simulink model "NLMPC_Acado_Deploy_Speedgoat"  (R2021b)
settings: Solver=ode4  StartTime=0.0  StopTime=250  FixedStep=Ts  RelTol=1e-3  EnableMultiTasking=on
InitFcn:
  | ts = 0.001;
  | sin_base_freq = 1;
  | ampl = 6;
values from neighbouring files (symbols this model uses):
  Ad = sysd.A    [ACADO_NMPC_Main_File.m]
  Bd = sysd.B    [ACADO_NMPC_Main_File.m]
  eta = 0.94    [ACADO_NMPC_Main_File.m]
  Fext = [0 -1808.57139 -3027.52429 -3695.96924 -3861.91987 -3579.58608 -2906.76949 -1902.55612 -625.46835 867.809323 2523.07436 4288.62667 ... (9001 elements, 9001x1)]    [Fext.mat]
  Fk = 13893.63    [ACADO_NMPC_Main_File.m]
  Ts = 0.1    [ACADO_NMPC_Main_File.m]
  Wh1 = 2*[0         0      -c11/2   0 ... (first row only)    [ACADO_NMPC_Main_File.m]
  Wh2 = 2*[0         0       0       0 ... (first row only)    [ACADO_NMPC_Main_File.m]
  Wh3 = 2*[0         0       0       0 ... (first row only)    [ACADO_NMPC_Main_File.m]
  Wh4 = 2*[0         0      -c11/2   0 ... (first row only)    [ACADO_NMPC_Main_File.m]
  WNmat = WN    [ACADO_NMPC_Main_File.m]
  yref = [y(:);yN(:)]    [ACADO_NMPC_Main_File.m]
undefined symbols (not defined in the file or in its folder): C, IO, Mode
libraries: simulink x1, speedgoatlib_IO754 x1, dspstat3 x1
settings Model: sg_rtwmakecfg_data=_sglibc__sg_netxLib_  Creator=lab  LastModifiedBy=z4q9r
settings SolverCC: ConcurrentTasks=on  AlgebraicLoopSolver=TrustRegion  PositivePriorityOrder=on  AutoInsertRateTranBlk=on  InsertRTBMode=Never (minimum delay)
settings DataIOCC: LimitDataPoints=on  SaveFormat=StructureWithTime  ReturnWorkspaceOutputs=off
settings OptimizationCC: BlockReduction=off  DefaultParameterBehavior=Inlined  OptimizeBlockIOStorage=off  BufferReuse=off  GlobalBufferReuse=off  ExpressionFolding=off  LocalBlockOutputs=off  OptimizeDataStoreBuffers=off  BusAssignmentInplaceUpdate=off
settings DebuggingCC: TasksWithSamePriorityMsg=none  UnconnectedInputMsg=none  UnconnectedOutputMsg=none  UnconnectedLineMsg=none  SFMachineParentedDataDiag=warning  ArithmeticOperatorsInVariantConditions=warning
settings HardwareCC: ProdBitPerLong=64  ProdLongLongMode=on  ProdHWDeviceType=Intel->x86-64 (Linux 64)
settings SFSimCC: SimUseLocalCustomCode=off  CustomCodeUndefinedFunction=UseInterfaceOnly
settings RTWCC: Description=Simulink Real-Time  SystemTargetFile=slrealtime.tlc  TemplateMakefile=slrealtime_default_tmf  RTWUseLocalCustomCode=off  CustomSource=Bounds.c Constraints.c Flipper.c Indexlist.c Matrices.c MessageHandling.c Options.c OQPinterface.c QProblem.c QProblemB.c Utils.c acado_solver.c acado_integrator.c acado_qpoases3_interface.c  Toolchain=Simulink Real-Time Toolchain  BuildConfiguration=Faster Runs  CodeExecutionProfiling=on  TargetLang=C++

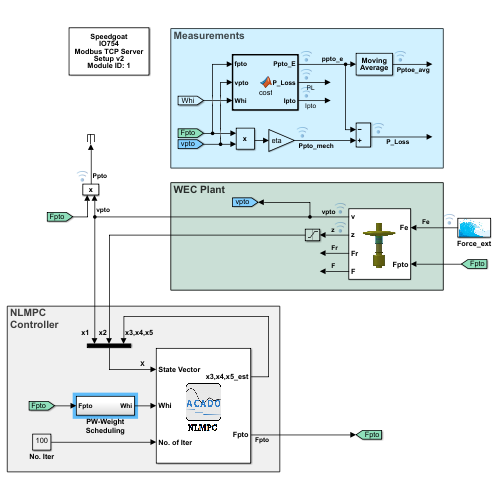
[thumbnail: Simulink's stored preview of the top-level diagram]
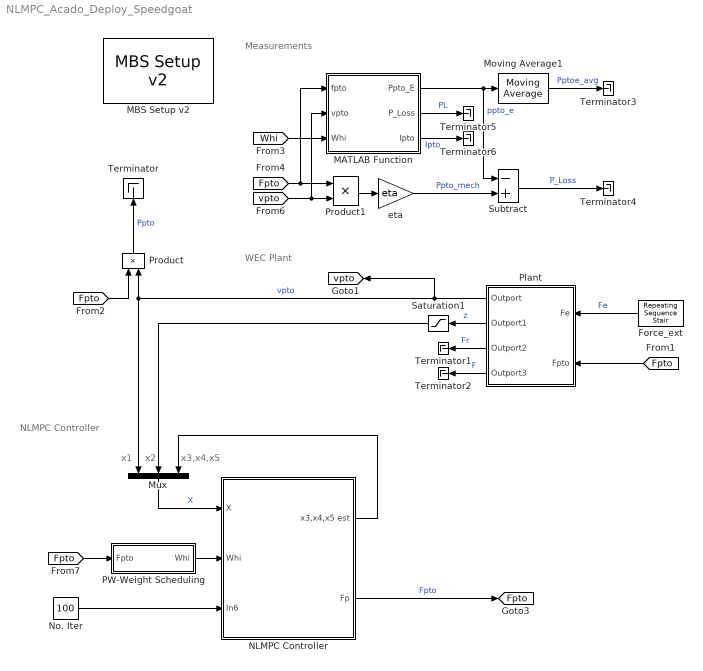
== system NLMPC_Acado_Deploy_Speedgoat ==
  note: x1
  note: x3,x4,x5
  note: x2
  note: NLMPC
      | Controller
  note: WEC Plant
  note: Measurements
  Force_ext : simulink/Sources/Repeating Sequence Stair  OutValues=Fext*1  tsamp=Ts  OutMin=[]  OutMax=[]  OutDataTypeStr=double  OutputDataTypeScalingMode=double  OutDataType=fixdt(0,8)  ConRadixGroup=Best Precision: Vector-wise  OutScaling=2^-12  mask(Repeating Sequence Stair){}
      mask Display:
      | % This is a new mask on top of the base mask.
      | % Use "View base mask" link below to see the base mask.
      | image('Image4.jpg')
  MATLAB Function : MATLAB Function  TreatAsAtomicUnit=on
  "MBS Setup v2 " : speedgoatlib_IO754/MBS Setup v2   id=1  drvLetter=C:  cfgMode=Warmstart  busSlot=-1  opMode=IO-Mode  busStart=Automatic  dataSwap=off  mapFC1FC3=off  serverCon=4  conWdgTime=1000  resTimeout=2000  sndAckTimeout=31000  conAckTimeout=31000  closeAckTimeout=13000  ipAdr=192.168.2.5  netmask=255.255.255.0  gateway=192.168.2.1  bootP=off  dhcp=off  enaMsgMode=off  coilStartAdr=0  coilQty=65536  descreteInputsStartAdr=0  descreteInputsQty=65536  holdingRegStartAdr=0  holdingRegQty=65536  inputRegStartAdr=0  inputRegQty=65536  blockInfo=setup_v2  speedgoatMainProtl=IO75X_IO64X  speedgoatSubProtl=IO754  protocolDescirption=Modbus TCP Server (slave)  filesBL="[\"1\", \"NETX100.BIN\"]"  filesFW="[\"1\", \"CIFXOMB.NXF\", \"2.6.0.6\", \"Open Modbus/TCP\"]"  filesCfg="[\"1\", \"INIBATCH.NXD\"]"  devData="[\"0000\", \"15CF\", \"0000\", \"0000\"]"  protocol=IO754  firmware=Modbus TCP Server
      settings: SourceProductName=Simulink Real-Time: Speedgoat I/O Driver Library
  Moving Average1 : dspstat3/Moving Average  Method=Sliding window  ForgettingFactorPort=off  SpecifyWindowLength=on  WindowLength=1000  ForgettingFactor=0.9  SimulateUsing=Code generation
  Mux : Mux  Inputs=3
  NLMPC Controller : Subsystem
      mask Display:
      | image('Image2.jpg')
      | port_label('input', 1, 'State Vector');
      | %port_label('input', 2, 'Ref');
      | port_label('input', 2, 'Whi');
      | %port_label('input', 4, 'WN');
      | %port_label('input', 5, 'Bounds');
      | %port_label('input', 6, 'Parameters');
      | port_label('input', 3, 'No. of Iter');
      | 
      | port_label('output', 1, 'x3,x4,x5_est');
      | port_label('output', 2, 'Fpto');
      | %port_label('output', 3, 'U Pred');
      | %port_label('output', 3, 'QP Status');
      | %port_label('output', 5, 'KKT Tol');
      | %port_label('output', 6, 'Fval');
  No. Iter : Constant  Value=100  OutDataTypeStr=double  SampleTime=Ts
  PW-Weight Scheduling : Subsystem
  Plant : Subsystem
      mask Display:
      | image('Image1.png')
      | 
      | port_label('input',2,'Fpto')
      | port_label('input',1,'Fe')
      | port_label('output',1,'v')
      | port_label('output',2,'z')
      | port_label('output',3,'Fr')
      | port_label('output',4,'F')
  Product : Product
  Product1 : Product
  Saturation1 : Saturate  UpperLimit=1.5  LowerLimit=-1.5
  Subtract : Sum  Inputs=-+
  Terminator{,1..6} (7 alike) : Terminator
  eta : Gain  Gain=eta
  tag scope: Fpto=global, vpto=global
  wires:
  Saturation1/1 -> Mux/2
  [Fpto] -> Product/1
  Product/1 -> Terminator/1  "Ppto"
  [Fpto] -> PW-Weight Scheduling/1(Fpto)
  No. Iter/1 -> NLMPC Controller/3(In6)
  NLMPC Controller/1(x3,x4,x5 est) -> Mux/3
  NLMPC Controller/2(Fp) -> [Fpto]  "Fpto"
  Mux/1 -> NLMPC Controller/1(X)  "X"
  PW-Weight Scheduling/1(Whi) -> NLMPC Controller/2(Whi)
  Plant/3(Outport2) -> Terminator1/1  "Fr"
  Plant/2(Outport1) -> Saturation1/1  "z"
  [Fpto] -> Plant/2(Fpto)
  Plant/4(Outport3) -> Terminator2/1  "F"
  Force_ext/1 -> Plant/1(Fe)  "Fe"
  Plant/1(Outport) -> Product/2, Mux/1, [vpto]  "vpto"
  [Whi] -> MATLAB Function/3(Whi)
  Moving Average1/1 -> Terminator3/1  "Pptoe_avg"
  MATLAB Function/2(P_Loss) -> Terminator5/1  "PL"
  Subtract/1 -> Terminator4/1  "P_Loss"
  Product1/1 -> eta/1
  MATLAB Function/1(Ppto_E) -> Subtract/1, Moving Average1/1  "ppto_e"
  MATLAB Function/3(Ipto) -> Terminator6/1  "Ipto"
  eta/1 -> Subtract/2  "Ppto_mech"
  [Fpto] -> Product1/1, MATLAB Function/1(fpto)
  [vpto] -> MATLAB Function/2(vpto), Product1/2

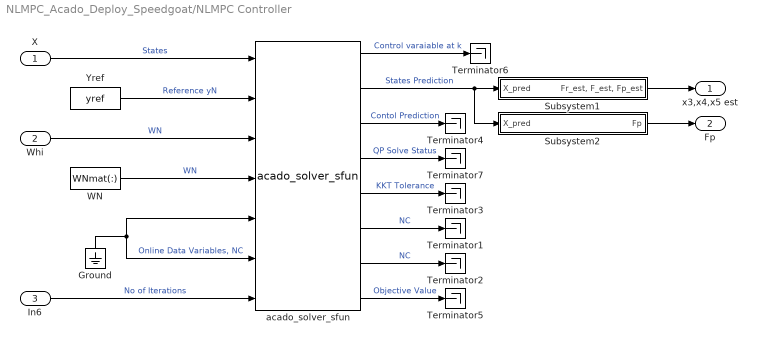
== system NLMPC_Acado_Deploy_Speedgoat/NLMPC Controller ==
  X : Inport
  Whi : Inport  Port=2
  In6 : Inport  Port=3
  Ground : Ground
  Subsystem1 : Subsystem
  Subsystem2 : Subsystem
  Terminator{1..7} (7 alike) : Terminator
  WN : Constant  Value=WNmat(:)  OutDataTypeStr=double  SampleTime=Ts
  Yref : Constant  Value=yref  OutDataTypeStr=double  SampleTime=Ts
  acado_solver_sfun : S-Function  FunctionName=acado_solver_sfun  Parameters=xInit, zInit, uInit, Wmat, WNmat, bValues  SFunctionDeploymentMode=off  EnableBusSupport=off  mask(Legacy Function){SFunctionSpec=acado_step(ACADOinput u1[1], ACADOoutput y1[1]), ShowSpec=off}
      mask prompts: ShowSpec "Display function specification"
      mask help:
      | This block allows you to call the legacy functions specified by the following Legacy Code Tool definition:
      | def.SFunctionName = 'acado_solver_sfun';
      | def.OutputFcnSpec = 'acado_step(ACADOinput u1[1], ACADOoutput y1[1])';
      | def.StartFcnSpec = 'acado_initialize( void )';
      | def.TerminateFcnSpec = 'acado_cleanup( void )';
      | def.HeaderFiles = {'acado_common.h', 'acado_solver_sfunction.h'};
      | def.SourceFiles = {'acado_solver.c', 'acado_integrator.c', 'acado_auxiliary_functions.c', 'acado_solver_sfunction.c', 'acado_qpoases_interface.cpp', 'qpoases/SRC/Bounds.cpp', 'qpoases/SRC/Constraints.cpp', 'qpoases/SRC/CyclingManager.cpp', 'qpoases/SRC/Indexlist.cpp', 'qpoases/SRC/MessageHandling.cpp', 'qpoases/SRC/QProblem.cpp', 'qpoases/SRC/QProblemB.cpp', 'qpoases/SRC/SubjectTo.cpp', 'qpoases/SRC/Utils.cpp', 'qpoases/SRC/EXTRAS/SolutionAnalysis.cpp'};
      | def.IncPaths = {'qpoases', 'qpoases/INCLUDE', 'qpoases/SRC'};
      | def.Options.language = 'C++';
      mask Help: <p>This block was generated automatically by the Legacy Code Tool. For detailed help on this tool, call<a href="matlab:legacy_code('help')"> legacy_code('help')</a>.</p>
      mask Callback ShowSpec:
      | if strcmp(get_param(gcbh, 'ShowSpec'), 'on')
      |   set_param(gcbh, 'MaskDisplay', sprintf('fprintf(''%s'');', get_param(gcbh, 'SFunctionSpec')));
      | else
      |   set_param(gcbh, 'MaskDisplay', sprintf('fprintf(''%s'');', get_param(gcbh, 'FunctionName')));
      | end
      mask Display: fprintf('acado_solver_sfun');
  x3,x4,x5 est : Outport  VectorParamsAs1DForOutWhenUnconnected=off
  Fp : Outport  Port=2  VectorParamsAs1DForOutWhenUnconnected=off
  wires:
  Ground/1 -> acado_solver_sfun/6, acado_solver_sfun/5  "Online Data Variables, NC"
  acado_solver_sfun/3 -> Terminator4/1  "Contol Prediction"
  acado_solver_sfun/1 -> Terminator6/1  "Control varaiable at k"
  In6/1 -> acado_solver_sfun/7  "No of Iterations"
  Yref/1 -> acado_solver_sfun/2  "Reference yN"
  acado_solver_sfun/4 -> Terminator7/1  "QP Solve Status"
  acado_solver_sfun/5 -> Terminator3/1  "KKT Tolerance"
  acado_solver_sfun/8 -> Terminator5/1  "Objective Value"
  WN/1 -> acado_solver_sfun/4  "WN"
  acado_solver_sfun/6 -> Terminator1/1  "NC"
  acado_solver_sfun/7 -> Terminator2/1  "NC"
  acado_solver_sfun/2 -> Subsystem2/1(X_pred), Subsystem1/1(X_pred)  "States Prediction"
  Subsystem1/1("Fr_est, F_est, Fp_est") -> x3,x4,x5 est/1
  X/1 -> acado_solver_sfun/1  "States"
  Subsystem2/1(Fp) -> Fp/1
  Whi/1 -> acado_solver_sfun/3  "WN"

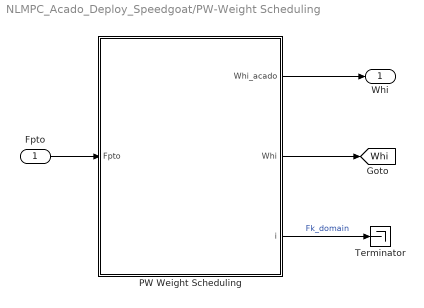
== system NLMPC_Acado_Deploy_Speedgoat/PW-Weight Scheduling ==
  Fpto : Inport
  PW Weight Scheduling : MATLAB Function  TreatAsAtomicUnit=on
  Terminator : Terminator
  Whi : Outport  VectorParamsAs1DForOutWhenUnconnected=off
  tag scope: Whi=global
  wires:
  PW Weight Scheduling/1(Whi_acado) -> Whi/1
  PW Weight Scheduling/3(i) -> Terminator/1  "Fk_domain"
  Fpto/1 -> PW Weight Scheduling/1(Fpto)
  PW Weight Scheduling/2(Whi) -> [Whi]

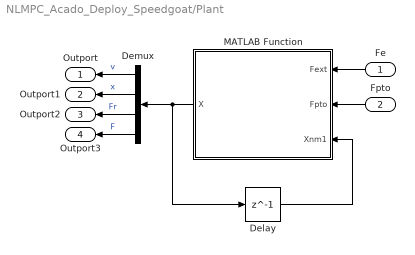
== system NLMPC_Acado_Deploy_Speedgoat/Plant ==
  Fe : Inport
  Fpto : Inport  Port=2
  Delay : Delay  DelayLength=1
  Demux : Demux
  MATLAB Function : MATLAB Function  TreatAsAtomicUnit=on
  Outport : Outport  VectorParamsAs1DForOutWhenUnconnected=off
  Outport1 : Outport  Port=2  VectorParamsAs1DForOutWhenUnconnected=off
  Outport2 : Outport  Port=3  VectorParamsAs1DForOutWhenUnconnected=off
  Outport3 : Outport  Port=4  VectorParamsAs1DForOutWhenUnconnected=off
  wires:
  Demux/1 -> Outport/1  "v"
  Demux/2 -> Outport1/1  "x"
  Demux/4 -> Outport3/1  "F"
  Demux/3 -> Outport2/1  "Fr"
  Fpto/1 -> MATLAB Function/2(Fpto)
  Delay/1 -> MATLAB Function/3(Xnm1)
  MATLAB Function/1(X) -> Demux/1, Delay/1
  Fe/1 -> MATLAB Function/1(Fext)

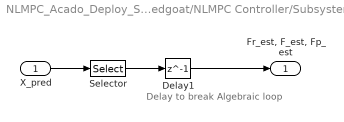
== system NLMPC_Acado_Deploy_Speedgoat/NLMPC Controller/Subsystem1 ==
  note: Delay to break
      | Algebraic loop
  X_pred : Inport
  Delay1 : Delay  DelayLength=1
  Selector : Selector  NumberOfDimensions=2  InputPortWidth=3  IndexOptions=Index vector (dialog),Index vector (dialog)  Indices=[2],[3 4 5]  OutputSizes=1,1
  "Fr_est, F_est, Fp_est" : Outport
  wires:
  Selector/1 -> Delay1/1
  X_pred/1 -> Selector/1
  Delay1/1 -> "Fr_est, F_est, Fp_est"/1

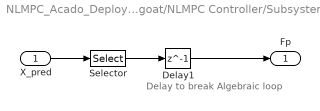
== system NLMPC_Acado_Deploy_Speedgoat/NLMPC Controller/Subsystem2 ==
  note: Delay to break
      | Algebraic loop
  X_pred : Inport
  Delay1 : Delay  DelayLength=1
  Selector : Selector  NumberOfDimensions=2  InputPortWidth=3  IndexOptions=Index vector (dialog),Index vector (dialog)  Indices=[1],[5]  OutputSizes=1,1
  Fp : Outport
  wires:
  Selector/1 -> Delay1/1
  X_pred/1 -> Selector/1
  Delay1/1 -> Fp/1

== matlab function NLMPC_Acado_Deploy_Speedgoat/MATLAB Function ==
  data: fpto input; vpto input; Ppto_E output; Whi input; Fk parameter; P_Loss output; Ipto output
function [Ppto_E,P_Loss,Ipto] = cost(fpto, vpto, Whi, Fk)
Ppto_E=-0.5*[fpto^2,fpto,vpto,1]*Whi*[fpto^2,fpto,vpto,1]';


c10=9.271331158e-1;
c11=2.986818189e-7;
c12=1.64275e-6;
c13=7.076786316e-2;
c14=1.385728e2;
c15=7.62150425e2;

c20=9.130091884e-1;
c21=1551/10448;

c30=9.669908116e-1;
c40=9.528668842e-1;
P_Loss=0;
Ipto=0;
%-----------------------------------
if(fpto <= -Fk)
P_Loss=(c10-0.94)*fpto*vpto+c11*fpto^2*vpto-c12*fpto^2+c13*fpto+c14*vpto-c15;
Ipto=(fpto-21539.45)/307.27;
end
%-----------------------------------
if(fpto > -Fk && fpto < 0 )
P_Loss=(c20-0.94)*fpto*vpto+c21*fpto;
Ipto=-sqrt(-fpto/1.0448);
end
%-----------------------------------
if(fpto >= 0 && fpto < Fk )
P_Loss=(c30-0.94)*fpto*vpto-c21*fpto;
Ipto=sqrt(fpto/1.0448);
end
%----------------------------------- 
if(fpto >= Fk )
P_Loss=(c40-0.94)*fpto*vpto+c11*fpto^2*vpto-c12*fpto^2-c13*fpto+c14*vpto-c15;
Ipto=sqrt(fpto/1.0448);
Ipto=(fpto+21539.45)/307.27;
end

P_Loss=-P_Loss;

%----------------------------------
end

% Negtive sign to converte minimization back to maximization
% 0.5 to cancel factor of 2 with Whi in ACADO main m-file
% when Npto>1, the effect is automatically taken ionto account by fp and Vp
% so no need to multiply W by Npto here.

== matlab function NLMPC_Acado_Deploy_Speedgoat/PW-Weight Scheduling/PW Weight Scheduling ==
  data: Fpto input; Whi_acado output; Whi output; i output; Wh1 parameter; Wh2 parameter; Wh3 parameter; Wh4 parameter; Fk parameter
function [Whi_acado,Whi,i]= Weight_Schedule(Fpto, Wh1, Wh2, Wh3, Wh4, Fk)
Whi=zeros(4);
i=0;
%-----------------------------------
if(Fpto <= -Fk)
    Whi=Wh1;
    i=1;
end
%-----------------------------------
if(Fpto > -Fk && Fpto < 0 )
    Whi=Wh2;
      i=2;
end
%-----------------------------------
if(Fpto >= 0 && Fpto < Fk )
    Whi=Wh3;
      i=3;
end
%----------------------------------- 
if(Fpto >= Fk )
    Whi=Wh4;
      i=4;
end

%-----------------------------------
Whi_acado=Whi(:);

end

== matlab function NLMPC_Acado_Deploy_Speedgoat/Plant/MATLAB Function ==
  data: Fext input size=1; Fpto input size=1; Xnm1 input size=[4 1]; Ad parameter size=[4 4]; X output size=[4 1]; Bd parameter size=[4 2]
function X = WECPlant(Fext,Fpto, Xnm1,Ad, Bd)

U=[Fpto Fext]'; % input vector
X=Ad*Xnm1+Bd*U; % state vector calculation from the previous state and input

end
